simulink model "Assignment4"  (R2014a)
settings: Solver=FixedStepDiscrete  StartTime=0.0  StopTime=300000  FixedStep=1  RelTol=1e-3
libraries: hdlsllib x15, simulink x10
settings Model: Creator=vu.du  LastModifiedBy=vu.du

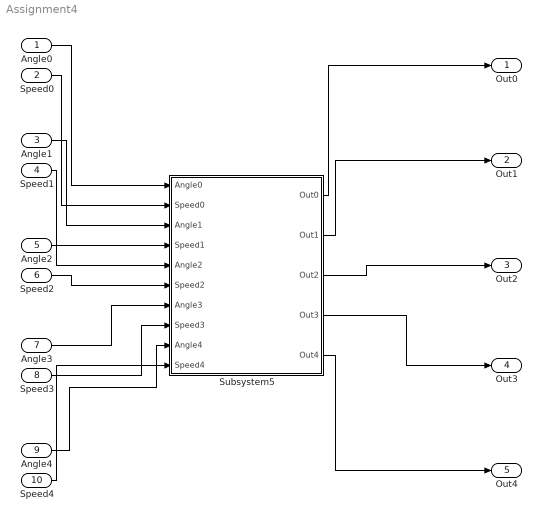
== system Assignment4 ==
  Angle0 : Inport  OutDataTypeStr=int8  SampleTime=1
  Speed0 : Inport  Port=2  OutDataTypeStr=int32  SampleTime=1
  Angle1 : Inport  Port=3  OutDataTypeStr=int8  SampleTime=1
  Speed1 : Inport  Port=4  OutDataTypeStr=int32  SampleTime=1
  Angle2 : Inport  Port=5  OutDataTypeStr=int8  SampleTime=1
  Speed2 : Inport  Port=6  OutDataTypeStr=int32  SampleTime=1
  Angle3 : Inport  Port=7  OutDataTypeStr=int8  SampleTime=1
  Speed3 : Inport  Port=8  OutDataTypeStr=int32  SampleTime=1
  Angle4 : Inport  Port=9  OutDataTypeStr=int8  SampleTime=1
  Speed4 : Inport  Port=10  OutDataTypeStr=int32  SampleTime=1
  Subsystem5 : Subsystem  TreatAsAtomicUnit=on
  Out0 : Outport
  Out1 : Outport  Port=2
  Out2 : Outport  Port=3
  Out3 : Outport  Port=4
  Out4 : Outport  Port=5
  wires:
  Angle0/1 -> Subsystem5/1(Angle0)
  Speed0/1 -> Subsystem5/2(Speed0)
  Angle1/1 -> Subsystem5/3(Angle1)
  Speed1/1 -> Subsystem5/4(Speed1)
  Angle2/1 -> Subsystem5/5(Angle2)
  Speed2/1 -> Subsystem5/6(Speed2)
  Angle3/1 -> Subsystem5/7(Angle3)
  Speed3/1 -> Subsystem5/8(Speed3)
  Angle4/1 -> Subsystem5/9(Angle4)
  Speed4/1 -> Subsystem5/10(Speed4)
  Subsystem5/1(Out0) -> Out0/1
  Subsystem5/2(Out1) -> Out1/1
  Subsystem5/3(Out2) -> Out2/1
  Subsystem5/4(Out3) -> Out3/1
  Subsystem5/5(Out4) -> Out4/1

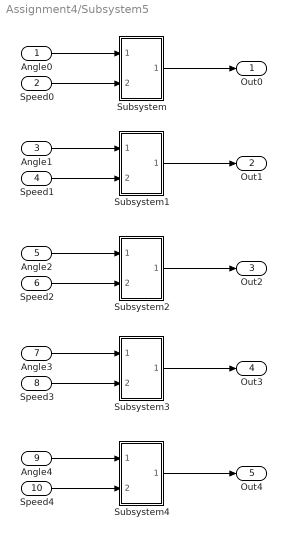
== system Assignment4/Subsystem5 ==
  Angle0 : Inport
  Speed0 : Inport  Port=2
  Angle1 : Inport  Port=3
  Speed1 : Inport  Port=4
  Angle2 : Inport  Port=5
  Speed2 : Inport  Port=6
  Angle3 : Inport  Port=7
  Speed3 : Inport  Port=8
  Angle4 : Inport  Port=9
  Speed4 : Inport  Port=10
  Subsystem : Subsystem
  Subsystem1 : Subsystem
  Subsystem2 : Subsystem
  Subsystem3 : Subsystem
  Subsystem4 : Subsystem
  Out0 : Outport
  Out1 : Outport  Port=2
  Out2 : Outport  Port=3
  Out3 : Outport  Port=4
  Out4 : Outport  Port=5
  wires:
  Subsystem/1(Out1) -> Out0/1
  Subsystem3/1(Out1) -> Out3/1
  Angle3/1 -> Subsystem3/1(Angle)
  Speed3/1 -> Subsystem3/2(Speed)
  Subsystem4/1(Out1) -> Out4/1
  Angle4/1 -> Subsystem4/1(Angle)
  Speed4/1 -> Subsystem4/2(Speed)
  Subsystem1/1(Out1) -> Out1/1
  Angle1/1 -> Subsystem1/1(Angle)
  Speed1/1 -> Subsystem1/2(Speed)
  Subsystem2/1(Out1) -> Out2/1
  Angle2/1 -> Subsystem2/1(Angle)
  Speed2/1 -> Subsystem2/2(Speed)
  Angle0/1 -> Subsystem/1(Angle)
  Speed0/1 -> Subsystem/2(Speed)

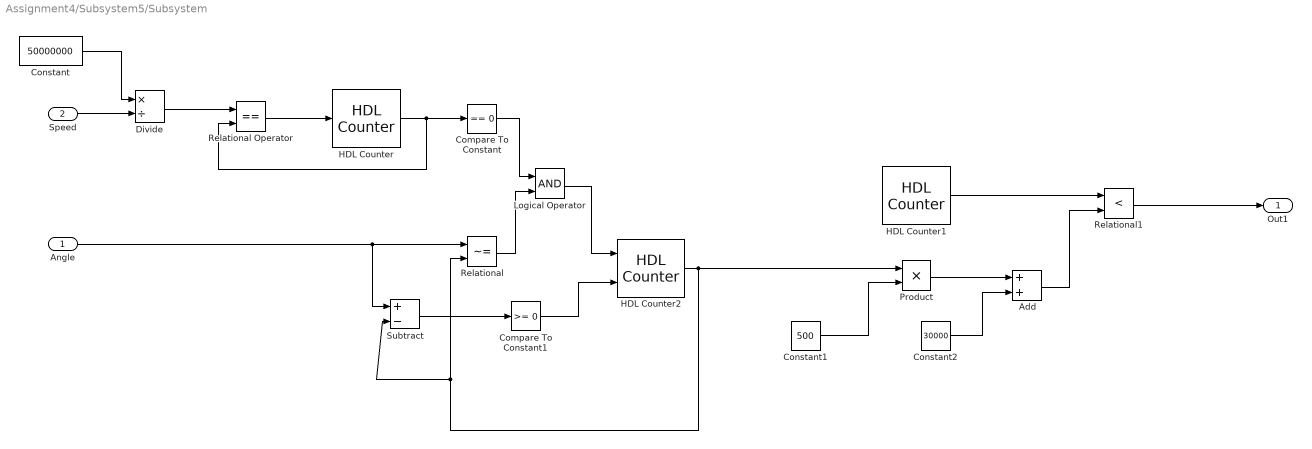
== system Assignment4/Subsystem5/Subsystem ==
  Angle : Inport
  Speed : Inport  Port=2
  Add : Sum
  Compare To Constant : simulink/Logic and Bit Operations/Compare To Constant  relop===  const=0  OutDataTypeStr=boolean
  Compare To Constant1 : simulink/Logic and Bit Operations/Compare To Constant  relop=>=  const=0  OutDataTypeStr=boolean
  Constant : Constant  Value=50000000  OutDataTypeStr=int32
  Constant1 : Constant  Value=500  OutDataTypeStr=int32
  Constant2 : Constant  Value=30000  OutDataTypeStr=int32
  Divide : Product  Inputs=*/  OutDataTypeStr=int32  SaturateOnIntegerOverflow=on  RndMeth=Zero
  HDL Counter : hdlsllib/HDL Operations/HDL Counter  CountType=Free running  CountInit=0  CountStep=1  CountMax=100  CountFromType=Initial value  CountFrom=0  CountResetPort=on  CountLoadPort=off  CountEnbPort=off  CountDirPort=off  CountDataType=Unsigned  CountWordLen=32  CountFracLen=0  CountSampTime=1
  HDL Counter1 : hdlsllib/HDL Operations/HDL Counter  CountType=Count limited  CountInit=0  CountStep=1  CountMax=1000000  CountFromType=Initial value  CountFrom=0  CountResetPort=off  CountLoadPort=off  CountEnbPort=off  CountDirPort=off  CountDataType=Unsigned  CountWordLen=32  CountFracLen=0  CountSampTime=1
  HDL Counter2 : hdlsllib/HDL Operations/HDL Counter  CountType=Count limited  CountInit=90  CountStep=1  CountMax=180  CountFromType=Specify  CountFrom=0  CountResetPort=off  CountLoadPort=off  CountEnbPort=on  CountDirPort=on  CountDataType=Unsigned  CountWordLen=32  CountFracLen=0  CountSampTime=1
  Logical Operator : Logic  AllPortsSameDT=off  OutDataTypeStr=boolean
  Product : Product
  Relational : RelationalOperator  Operator=~=  OutDataTypeStr=boolean
  Relational Operator : RelationalOperator  Operator===  OutDataTypeStr=boolean
  Relational1 : RelationalOperator  Operator=<  OutDataTypeStr=boolean
  Subtract : Sum  Inputs=+-
  Out1 : Outport
  wires:
  Relational/1 -> Logical Operator/2
  Divide/1 -> Relational Operator/1
  HDL Counter/1 -> Relational Operator/2, Compare To Constant/1
  Constant/1 -> Divide/1
  Speed/1 -> Divide/2
  Relational Operator/1 -> HDL Counter/1
  Subtract/1 -> Compare To Constant1/1
  Product/1 -> Add/1
  Compare To Constant1/1 -> HDL Counter2/2
  Constant2/1 -> Add/2
  Add/1 -> Relational1/2
  HDL Counter2/1 -> Product/1, Subtract/2, Relational/2
  Relational1/1 -> Out1/1
  Logical Operator/1 -> HDL Counter2/1
  Compare To Constant/1 -> Logical Operator/1
  HDL Counter1/1 -> Relational1/1
  Angle/1 -> Subtract/1, Relational/1
  Constant1/1 -> Product/2

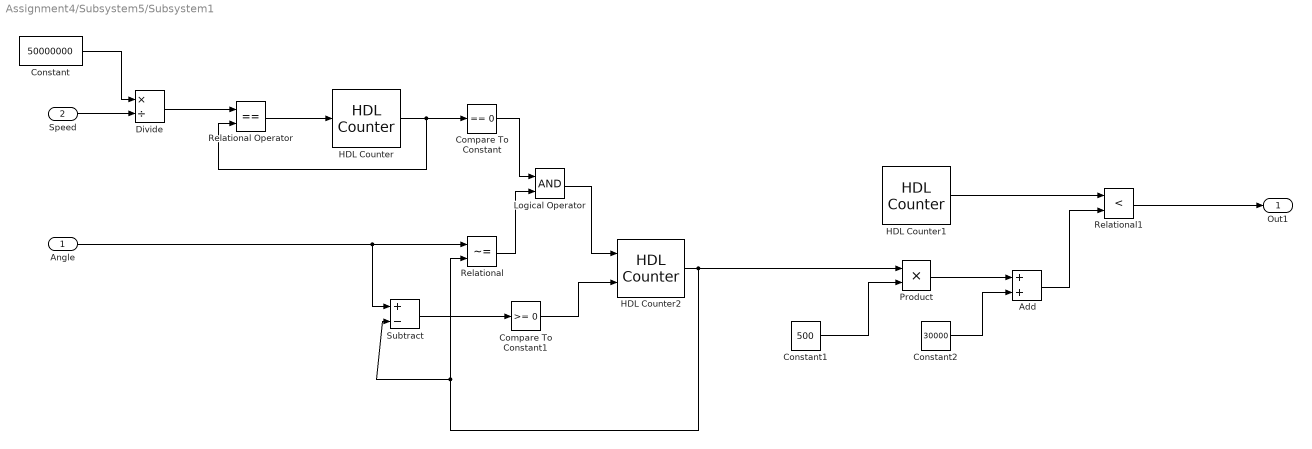
== system Assignment4/Subsystem5/Subsystem1 ==
  Angle : Inport
  Speed : Inport  Port=2
  Add : Sum
  Compare To Constant : simulink/Logic and Bit Operations/Compare To Constant  relop===  const=0  OutDataTypeStr=boolean
  Compare To Constant1 : simulink/Logic and Bit Operations/Compare To Constant  relop=>=  const=0  OutDataTypeStr=boolean
  Constant : Constant  Value=50000000  OutDataTypeStr=int32
  Constant1 : Constant  Value=500  OutDataTypeStr=int32
  Constant2 : Constant  Value=30000  OutDataTypeStr=int32
  Divide : Product  Inputs=*/  OutDataTypeStr=int32  SaturateOnIntegerOverflow=on  RndMeth=Zero
  HDL Counter : hdlsllib/HDL Operations/HDL Counter  CountType=Free running  CountInit=0  CountStep=1  CountMax=100  CountFromType=Initial value  CountFrom=0  CountResetPort=on  CountLoadPort=off  CountEnbPort=off  CountDirPort=off  CountDataType=Unsigned  CountWordLen=32  CountFracLen=0  CountSampTime=1
  HDL Counter1 : hdlsllib/HDL Operations/HDL Counter  CountType=Count limited  CountInit=0  CountStep=1  CountMax=1000000  CountFromType=Initial value  CountFrom=0  CountResetPort=off  CountLoadPort=off  CountEnbPort=off  CountDirPort=off  CountDataType=Unsigned  CountWordLen=32  CountFracLen=0  CountSampTime=1
  HDL Counter2 : hdlsllib/HDL Operations/HDL Counter  CountType=Count limited  CountInit=90  CountStep=1  CountMax=180  CountFromType=Specify  CountFrom=0  CountResetPort=off  CountLoadPort=off  CountEnbPort=on  CountDirPort=on  CountDataType=Unsigned  CountWordLen=32  CountFracLen=0  CountSampTime=1
  Logical Operator : Logic  AllPortsSameDT=off  OutDataTypeStr=boolean
  Product : Product
  Relational : RelationalOperator  Operator=~=  OutDataTypeStr=boolean
  Relational Operator : RelationalOperator  Operator===  OutDataTypeStr=boolean
  Relational1 : RelationalOperator  Operator=<  OutDataTypeStr=boolean
  Subtract : Sum  Inputs=+-
  Out1 : Outport
  wires:
  Relational/1 -> Logical Operator/2
  Divide/1 -> Relational Operator/1
  HDL Counter/1 -> Relational Operator/2, Compare To Constant/1
  Constant/1 -> Divide/1
  Speed/1 -> Divide/2
  Relational Operator/1 -> HDL Counter/1
  Subtract/1 -> Compare To Constant1/1
  Product/1 -> Add/1
  Compare To Constant1/1 -> HDL Counter2/2
  Constant2/1 -> Add/2
  Add/1 -> Relational1/2
  HDL Counter2/1 -> Product/1, Subtract/2, Relational/2
  Relational1/1 -> Out1/1
  Logical Operator/1 -> HDL Counter2/1
  Compare To Constant/1 -> Logical Operator/1
  HDL Counter1/1 -> Relational1/1
  Angle/1 -> Subtract/1, Relational/1
  Constant1/1 -> Product/2

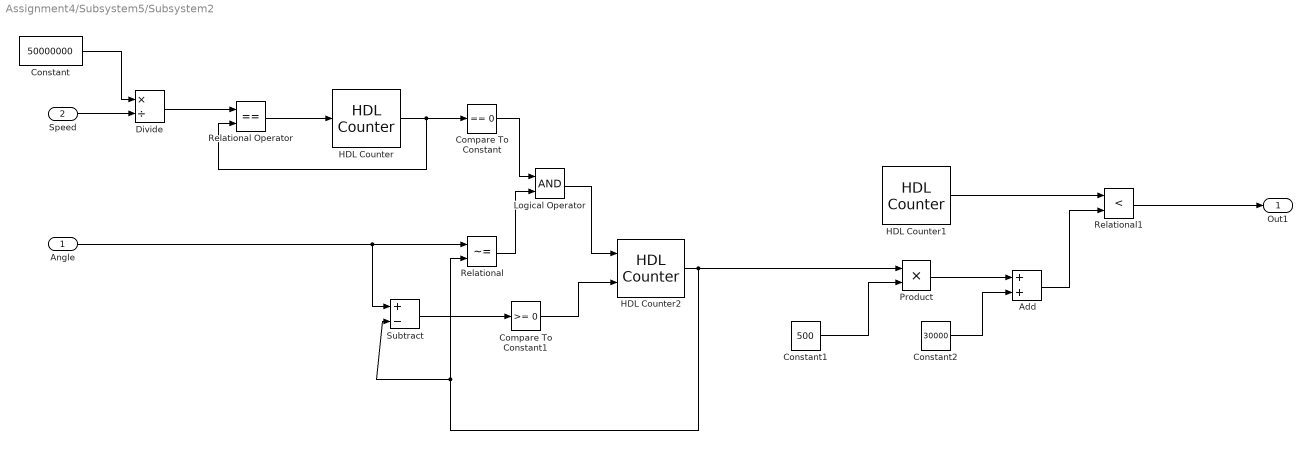
== system Assignment4/Subsystem5/Subsystem2 ==
  Angle : Inport
  Speed : Inport  Port=2
  Add : Sum
  Compare To Constant : simulink/Logic and Bit Operations/Compare To Constant  relop===  const=0  OutDataTypeStr=boolean
  Compare To Constant1 : simulink/Logic and Bit Operations/Compare To Constant  relop=>=  const=0  OutDataTypeStr=boolean
  Constant : Constant  Value=50000000  OutDataTypeStr=int32
  Constant1 : Constant  Value=500  OutDataTypeStr=int32
  Constant2 : Constant  Value=30000  OutDataTypeStr=int32
  Divide : Product  Inputs=*/  OutDataTypeStr=int32  SaturateOnIntegerOverflow=on  RndMeth=Zero
  HDL Counter : hdlsllib/HDL Operations/HDL Counter  CountType=Free running  CountInit=0  CountStep=1  CountMax=100  CountFromType=Initial value  CountFrom=0  CountResetPort=on  CountLoadPort=off  CountEnbPort=off  CountDirPort=off  CountDataType=Unsigned  CountWordLen=32  CountFracLen=0  CountSampTime=1
  HDL Counter1 : hdlsllib/HDL Operations/HDL Counter  CountType=Count limited  CountInit=0  CountStep=1  CountMax=1000000  CountFromType=Initial value  CountFrom=0  CountResetPort=off  CountLoadPort=off  CountEnbPort=off  CountDirPort=off  CountDataType=Unsigned  CountWordLen=32  CountFracLen=0  CountSampTime=1
  HDL Counter2 : hdlsllib/HDL Operations/HDL Counter  CountType=Count limited  CountInit=90  CountStep=1  CountMax=180  CountFromType=Specify  CountFrom=0  CountResetPort=off  CountLoadPort=off  CountEnbPort=on  CountDirPort=on  CountDataType=Unsigned  CountWordLen=32  CountFracLen=0  CountSampTime=1
  Logical Operator : Logic  AllPortsSameDT=off  OutDataTypeStr=boolean
  Product : Product
  Relational : RelationalOperator  Operator=~=  OutDataTypeStr=boolean
  Relational Operator : RelationalOperator  Operator===  OutDataTypeStr=boolean
  Relational1 : RelationalOperator  Operator=<  OutDataTypeStr=boolean
  Subtract : Sum  Inputs=+-
  Out1 : Outport
  wires:
  Relational/1 -> Logical Operator/2
  Divide/1 -> Relational Operator/1
  HDL Counter/1 -> Relational Operator/2, Compare To Constant/1
  Constant/1 -> Divide/1
  Speed/1 -> Divide/2
  Relational Operator/1 -> HDL Counter/1
  Subtract/1 -> Compare To Constant1/1
  Product/1 -> Add/1
  Compare To Constant1/1 -> HDL Counter2/2
  Constant2/1 -> Add/2
  Add/1 -> Relational1/2
  HDL Counter2/1 -> Product/1, Subtract/2, Relational/2
  Relational1/1 -> Out1/1
  Logical Operator/1 -> HDL Counter2/1
  Compare To Constant/1 -> Logical Operator/1
  HDL Counter1/1 -> Relational1/1
  Angle/1 -> Subtract/1, Relational/1
  Constant1/1 -> Product/2

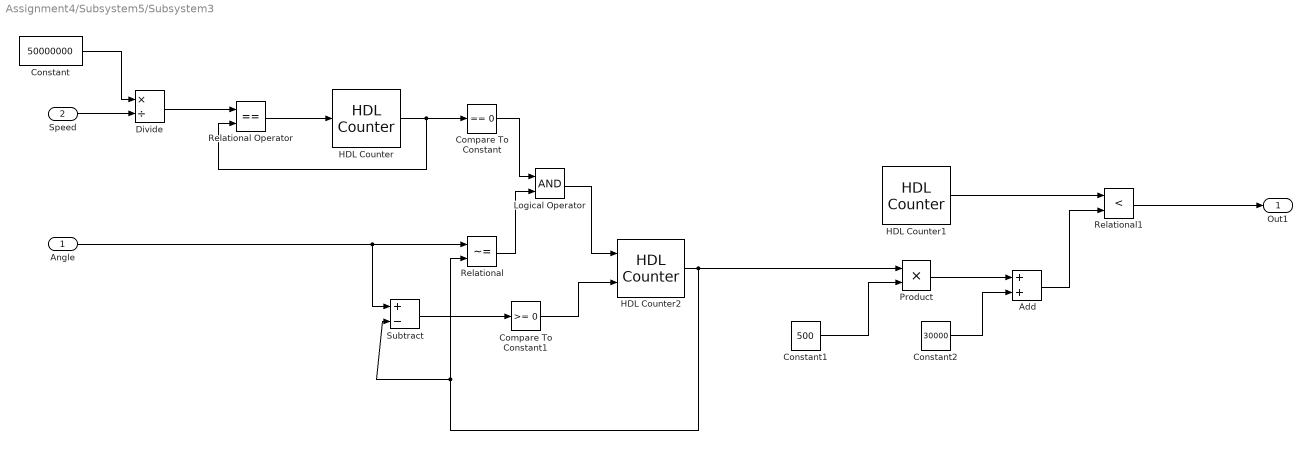
== system Assignment4/Subsystem5/Subsystem3 ==
  Angle : Inport
  Speed : Inport  Port=2
  Add : Sum
  Compare To Constant : simulink/Logic and Bit Operations/Compare To Constant  relop===  const=0  OutDataTypeStr=boolean
  Compare To Constant1 : simulink/Logic and Bit Operations/Compare To Constant  relop=>=  const=0  OutDataTypeStr=boolean
  Constant : Constant  Value=50000000  OutDataTypeStr=int32
  Constant1 : Constant  Value=500  OutDataTypeStr=int32
  Constant2 : Constant  Value=30000  OutDataTypeStr=int32
  Divide : Product  Inputs=*/  OutDataTypeStr=int32  SaturateOnIntegerOverflow=on  RndMeth=Zero
  HDL Counter : hdlsllib/HDL Operations/HDL Counter  CountType=Free running  CountInit=0  CountStep=1  CountMax=100  CountFromType=Initial value  CountFrom=0  CountResetPort=on  CountLoadPort=off  CountEnbPort=off  CountDirPort=off  CountDataType=Unsigned  CountWordLen=32  CountFracLen=0  CountSampTime=1
  HDL Counter1 : hdlsllib/HDL Operations/HDL Counter  CountType=Count limited  CountInit=0  CountStep=1  CountMax=1000000  CountFromType=Initial value  CountFrom=0  CountResetPort=off  CountLoadPort=off  CountEnbPort=off  CountDirPort=off  CountDataType=Unsigned  CountWordLen=32  CountFracLen=0  CountSampTime=1
  HDL Counter2 : hdlsllib/HDL Operations/HDL Counter  CountType=Count limited  CountInit=90  CountStep=1  CountMax=180  CountFromType=Specify  CountFrom=0  CountResetPort=off  CountLoadPort=off  CountEnbPort=on  CountDirPort=on  CountDataType=Unsigned  CountWordLen=32  CountFracLen=0  CountSampTime=1
  Logical Operator : Logic  AllPortsSameDT=off  OutDataTypeStr=boolean
  Product : Product
  Relational : RelationalOperator  Operator=~=  OutDataTypeStr=boolean
  Relational Operator : RelationalOperator  Operator===  OutDataTypeStr=boolean
  Relational1 : RelationalOperator  Operator=<  OutDataTypeStr=boolean
  Subtract : Sum  Inputs=+-
  Out1 : Outport
  wires:
  Relational/1 -> Logical Operator/2
  Divide/1 -> Relational Operator/1
  HDL Counter/1 -> Relational Operator/2, Compare To Constant/1
  Constant/1 -> Divide/1
  Speed/1 -> Divide/2
  Relational Operator/1 -> HDL Counter/1
  Subtract/1 -> Compare To Constant1/1
  Product/1 -> Add/1
  Compare To Constant1/1 -> HDL Counter2/2
  Constant2/1 -> Add/2
  Add/1 -> Relational1/2
  HDL Counter2/1 -> Product/1, Subtract/2, Relational/2
  Relational1/1 -> Out1/1
  Logical Operator/1 -> HDL Counter2/1
  Compare To Constant/1 -> Logical Operator/1
  HDL Counter1/1 -> Relational1/1
  Angle/1 -> Subtract/1, Relational/1
  Constant1/1 -> Product/2

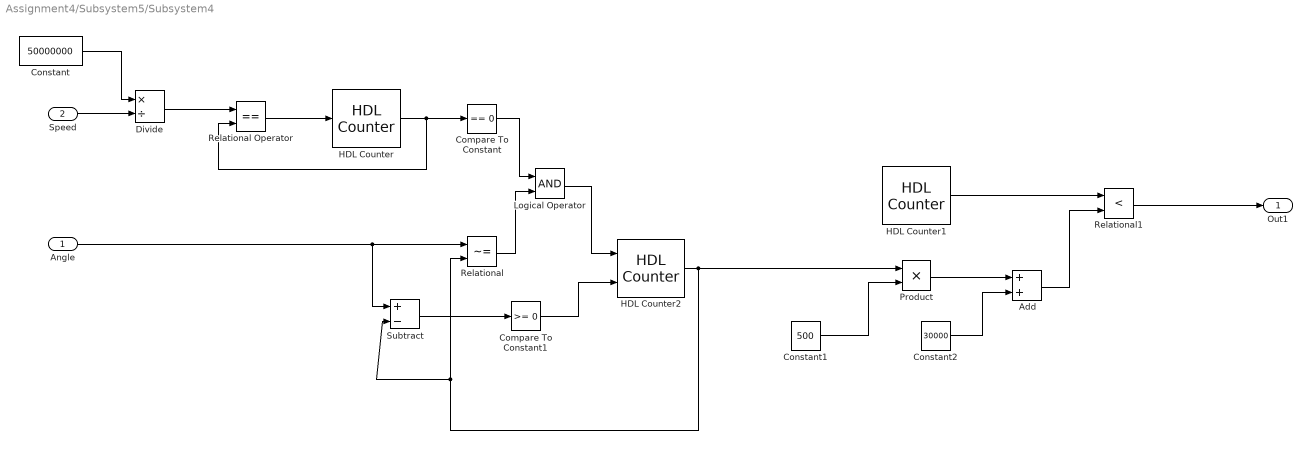
== system Assignment4/Subsystem5/Subsystem4 ==
  Angle : Inport
  Speed : Inport  Port=2
  Add : Sum
  Compare To Constant : simulink/Logic and Bit Operations/Compare To Constant  relop===  const=0  OutDataTypeStr=boolean
  Compare To Constant1 : simulink/Logic and Bit Operations/Compare To Constant  relop=>=  const=0  OutDataTypeStr=boolean
  Constant : Constant  Value=50000000  OutDataTypeStr=int32
  Constant1 : Constant  Value=500  OutDataTypeStr=int32
  Constant2 : Constant  Value=30000  OutDataTypeStr=int32
  Divide : Product  Inputs=*/  OutDataTypeStr=int32  SaturateOnIntegerOverflow=on  RndMeth=Zero
  HDL Counter : hdlsllib/HDL Operations/HDL Counter  CountType=Free running  CountInit=0  CountStep=1  CountMax=100  CountFromType=Initial value  CountFrom=0  CountResetPort=on  CountLoadPort=off  CountEnbPort=off  CountDirPort=off  CountDataType=Unsigned  CountWordLen=32  CountFracLen=0  CountSampTime=1
  HDL Counter1 : hdlsllib/HDL Operations/HDL Counter  CountType=Count limited  CountInit=0  CountStep=1  CountMax=1000000  CountFromType=Initial value  CountFrom=0  CountResetPort=off  CountLoadPort=off  CountEnbPort=off  CountDirPort=off  CountDataType=Unsigned  CountWordLen=32  CountFracLen=0  CountSampTime=1
  HDL Counter2 : hdlsllib/HDL Operations/HDL Counter  CountType=Count limited  CountInit=90  CountStep=1  CountMax=180  CountFromType=Specify  CountFrom=0  CountResetPort=off  CountLoadPort=off  CountEnbPort=on  CountDirPort=on  CountDataType=Unsigned  CountWordLen=32  CountFracLen=0  CountSampTime=1
  Logical Operator : Logic  AllPortsSameDT=off  OutDataTypeStr=boolean
  Product : Product
  Relational : RelationalOperator  Operator=~=  OutDataTypeStr=boolean
  Relational Operator : RelationalOperator  Operator===  OutDataTypeStr=boolean
  Relational1 : RelationalOperator  Operator=<  OutDataTypeStr=boolean
  Subtract : Sum  Inputs=+-
  Out1 : Outport
  wires:
  Relational/1 -> Logical Operator/2
  Divide/1 -> Relational Operator/1
  HDL Counter/1 -> Relational Operator/2, Compare To Constant/1
  Constant/1 -> Divide/1
  Speed/1 -> Divide/2
  Relational Operator/1 -> HDL Counter/1
  Subtract/1 -> Compare To Constant1/1
  Product/1 -> Add/1
  Compare To Constant1/1 -> HDL Counter2/2
  Constant2/1 -> Add/2
  Add/1 -> Relational1/2
  HDL Counter2/1 -> Product/1, Subtract/2, Relational/2
  Relational1/1 -> Out1/1
  Logical Operator/1 -> HDL Counter2/1
  Compare To Constant/1 -> Logical Operator/1
  HDL Counter1/1 -> Relational1/1
  Angle/1 -> Subtract/1, Relational/1
  Constant1/1 -> Product/2
